simulink model "ACC"  (R2025b)
settings: Solver=VariableStepAuto  StartTime=0.0  StopTime=10.0  RelTol=1e-3
settings Model: DataDictionary=ACC.sldd  Creator=vmari  LastModifiedBy=spadhi

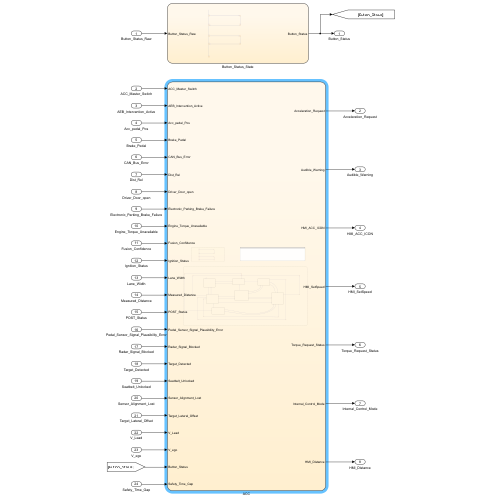
[thumbnail: Simulink's stored preview of the top-level diagram]
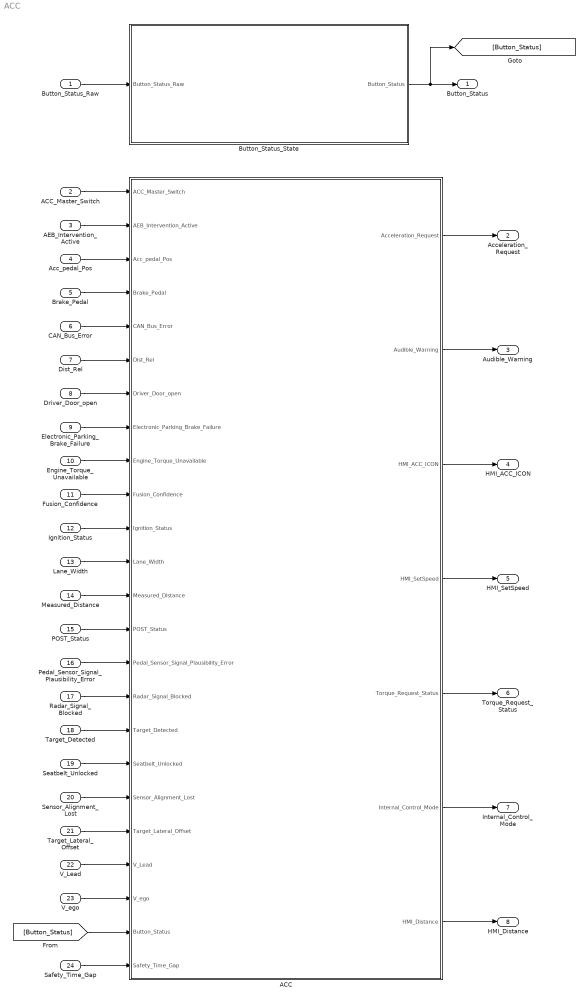
== system ACC ==
  Button_Status_Raw : Inport
  ACC_Master_Switch : Inport  Port=2
  AEB_Intervention_Active : Inport  Port=3
  Acc_pedal_Pos : Inport  Port=4
  Brake_Pedal : Inport  Port=5
  CAN_Bus_Error : Inport  Port=6
  Dist_Rel : Inport  Port=7
  Driver_Door_open : Inport  Port=8
  Electronic_Parking_Brake_Failure : Inport  Port=9
  Engine_Torque_Unavailable : Inport  Port=10
  Fusion_Confidence : Inport  Port=11
  Ignition_Status : Inport  Port=12
  Lane_Width : Inport  Port=13
  Measured_Distance : Inport  Port=14
  POST_Status : Inport  Port=15
  Pedal_Sensor_Signal_Plausibility_Error : Inport  Port=16
  Radar_Signal_Blocked : Inport  Port=17
  Target_Detected : Inport  Port=18
  Seatbelt_Unlocked : Inport  Port=19
  Sensor_Alignment_Lost : Inport  Port=20
  Target_Lateral_Offset : Inport  Port=21
  V_Lead : Inport  Port=22
  V_ego : Inport  Port=23
  Safety_Time_Gap : Inport  Port=24
  ACC : Stateflow chart  TreatAsAtomicUnit=on
  Button_Status_State : Stateflow chart  TreatAsAtomicUnit=on
  Button_Status : Outport
  Acceleration_Request : Outport  Port=2
  Audible_Warning : Outport  Port=3
  HMI_ACC_ICON : Outport  Port=4
  HMI_SetSpeed : Outport  Port=5
  Torque_Request_Status : Outport  Port=6
  Internal_Control_Mode : Outport  Port=7
  HMI_Distance : Outport  Port=8
  wires:
  Button_Status_Raw/1 -> Button_Status_State/1(Button_Status_Raw)
  Button_Status_State/1(Button_Status) -> [Button_Status], Button_Status/1
  [Button_Status] -> ACC/23(Button_Status)
  ACC_Master_Switch/1 -> ACC/1(ACC_Master_Switch)
  AEB_Intervention_Active/1 -> ACC/2(AEB_Intervention_Active)
  Acc_pedal_Pos/1 -> ACC/3(Acc_pedal_Pos)
  Brake_Pedal/1 -> ACC/4(Brake_Pedal)
  CAN_Bus_Error/1 -> ACC/5(CAN_Bus_Error)
  Driver_Door_open/1 -> ACC/7(Driver_Door_open)
  Electronic_Parking_Brake_Failure/1 -> ACC/8(Electronic_Parking_Brake_Failure)
  Engine_Torque_Unavailable/1 -> ACC/9(Engine_Torque_Unavailable)
  Fusion_Confidence/1 -> ACC/10(Fusion_Confidence)
  Ignition_Status/1 -> ACC/11(Ignition_Status)
  Dist_Rel/1 -> ACC/6(Dist_Rel)
  Lane_Width/1 -> ACC/12(Lane_Width)
  Measured_Distance/1 -> ACC/13(Measured_Distance)
  POST_Status/1 -> ACC/14(POST_Status)
  Pedal_Sensor_Signal_Plausibility_Error/1 -> ACC/15(Pedal_Sensor_Signal_Plausibility_Error)
  Radar_Signal_Blocked/1 -> ACC/16(Radar_Signal_Blocked)
  Target_Detected/1 -> ACC/17(Target_Detected)
  Seatbelt_Unlocked/1 -> ACC/18(Seatbelt_Unlocked)
  Sensor_Alignment_Lost/1 -> ACC/19(Sensor_Alignment_Lost)
  Target_Lateral_Offset/1 -> ACC/20(Target_Lateral_Offset)
  Safety_Time_Gap/1 -> ACC/24(Safety_Time_Gap)
  V_ego/1 -> ACC/22(V_ego)
  V_Lead/1 -> ACC/21(V_Lead)
  ACC/1(Acceleration_Request) -> Acceleration_Request/1
  ACC/2(Audible_Warning) -> Audible_Warning/1
  ACC/3(HMI_ACC_ICON) -> HMI_ACC_ICON/1
  ACC/4(HMI_SetSpeed) -> HMI_SetSpeed/1
  ACC/5(Torque_Request_Status) -> Torque_Request_Status/1
  ACC/6(Internal_Control_Mode) -> Internal_Control_Mode/1
  ACC/7(HMI_Distance) -> HMI_Distance/1

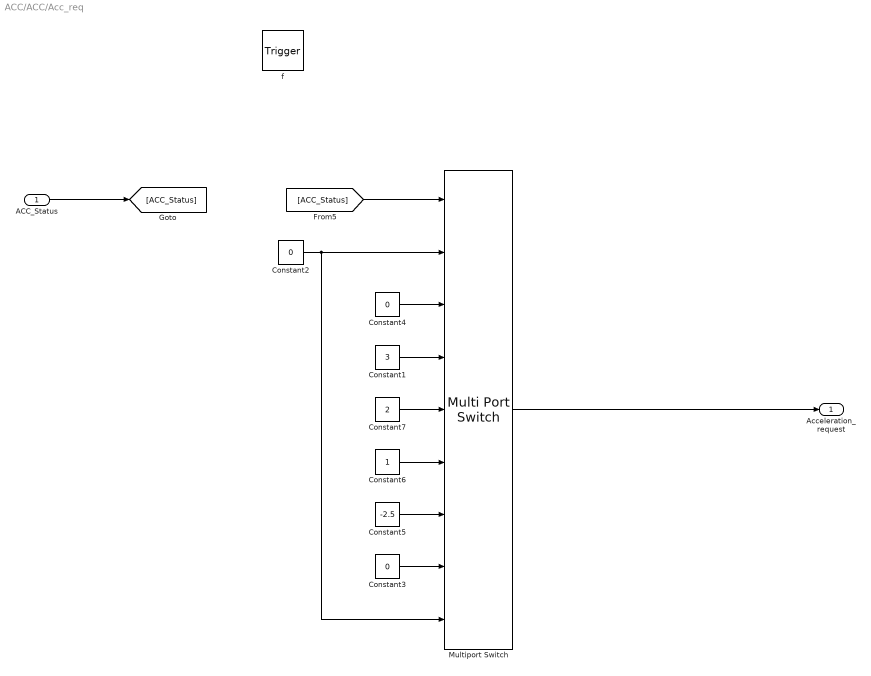
== system ACC/ACC/Acc_req ==
  ACC_Status : Inport  OutDataTypeStr=double  PortDimensions=1
  f : TriggerPort  TriggerType=function-call  VariantControl=(inherit)  SampleTime=0.01
      settings: CopyFcn=Stateflow.SLINSF.SimulinkMan.removeBlockPreDeleteFcn  PreDeleteFcn=Stateflow.SLINSF.SimulinkMan.unsafePredeleteFcn
  Constant1 : Constant  Value=3
  Constant2 : Constant  Value=0
  Constant3 : Constant  Value=0
  Constant4 : Constant  Value=0
  Constant5 : Constant  Value=-2.5
  Constant6 : Constant
  Constant7 : Constant  Value=2
  Multiport Switch : MultiPortSwitch  DataPortOrder=Zero-based contiguous  Inputs=7  DataPortForDefault=Additional data port  zeroidx=on  SaturateOnIntegerOverflow=off  InputSameDT=off
  Acceleration_request : Outport
  wires:
  ACC_Status/1 -> [ACC_Status]
  [ACC_Status] -> Multiport Switch/1
  Constant2/1 -> Multiport Switch/9, Multiport Switch/2
  Constant3/1 -> Multiport Switch/8
  Constant4/1 -> Multiport Switch/3
  Constant5/1 -> Multiport Switch/7
  Multiport Switch/1 -> Acceleration_request/1
  Constant1/1 -> Multiport Switch/4
  Constant7/1 -> Multiport Switch/5
  Constant6/1 -> Multiport Switch/6

== stateflow chart ACC/Button_Status_State ==
  (default) -> (junction 29)
  (junction 29) -> (junction 4) [order 1] : [Button_Status_Raw == 1]
  (junction 29) -> (junction 8) [order 2]
  (junction 4) -> (junction 6) : {Button_Status = Dt_Enum_Button_Status_E.SET}
  (junction 6) -> (junction 8)
  (junction 8) -> (junction 11)
  (junction 11) -> (junction 13) [order 1] : [Button_Status_Raw == 2]
  (junction 11) -> (junction 17) [order 2]
  (junction 13) -> (junction 15) : {Button_Status = Dt_Enum_Button_Status_E.CANCEL}
  (junction 15) -> (junction 17)
  (junction 17) -> (junction 20) : {Button_Status = Dt_Enum_Button_Status_E.NONE}
  data: Button_Status_Raw input; Button_Status output Enum: Dt_Enum_Button_Status_E

== stateflow chart ACC/ACC ==
  state Set_Speed_Controller [parallel]
    settings: executionOrder=2
    (default) -> (junction 162)
    (junction 162) -> (junction 165) [order 1] : [Target_Detected == true]
    (junction 162) -> (junction 164) [order 2]
    (junction 165) -> (junction 168) : {V_set = V_Lead}
    (junction 168) -> (junction 164)
    (junction 164) -> (junction 171)
    (junction 171) -> (junction 173) [order 1] : [Target_Detected == false && Button_Status ==Dt_Enum_Button_Status_E.SET ]
    (junction 171) -> (junction 176) [order 2]
    (junction 173) -> (junction 175) : {V_set = V_ego}
    (junction 175) -> (junction 176)
  state Acceleration_request = Acc_req(ACC_Status) [function]
  state ACC_States [parallel]
    settings: executionOrder=1
    state ACC_Off
      en:
      ACC_Status = 0;
      du:
      Acceleration_Request = Acc_req(ACC_Status);
      Torque_Request_Status = Disabled;
      HMI_ACC_ICON = Off;
      HMI_SetSpeed = V_set;
      Audible_Warning = None;
      Internal_Control_Mode = Standstill;
    state ACC_Fault
      ACC_Status = 2;
      Acceleration_Request = Acc_req(ACC_Status);
      %Rampto0
      Torque_Request_Status = Fault;
      HMI_ACC_ICON = Red;
      Audible_Warning = Loud_Chime;
      Internal_Control_Mode = Error;
    state ACC_Override
      en:
      ACC_Status = 6;
      du:
      Acceleration_Request = Acc_req(ACC_Status);
      Torque_Request_Status = Override;
      HMI_ACC_ICON = Blink_Green;
      Audible_Warning = Chime;%V>Vset for x
      Internal_Control_Mode = Passive;
    state ACC_Active
      ACC_Status = 3;
      Acceleration_Request = Acc_req(ACC_Status);
      %Vset-Vego
      Torque_Request_Status = Longi;
      HMI_ACC_ICON = Green;
      HMI_SetSpeed = 0;%Current_SetSpeed
      Audible_Warning = Single_Beep;
      Internal_Control_Mode = Speedctrl;
    state ACC_Active_Follow
      ACC_Status = 4;
      Acceleration_Request = Acc_req(ACC_Status);
      %Drel Cal
      Torque_Request_Status = Dis_active;
      HMI_ACC_ICON = Green;
      HMI_Distance = 1;%1-5 Bars
      Audible_Warning = None;
      Internal_Control_Mode = Distctrl;
    state ACC_Stanby
      en:
      ACC_Status = 1;
      du:
      Acceleration_Request = Acc_req(ACC_Status);
      Torque_Request_Status = Standby;
      HMI_ACC_ICON = White;
      HMI_SetSpeed = 0;%Prev Speed
      Audible_Warning = None;
      Internal_Control_Mode = Monitoring;
    state ACC_Stop_Hold
      en:
      ACC_Status = 5;
      du:
      Acceleration_Request = Acc_req(ACC_Status);
      Torque_Request_Status = Hold_Req;
      HMI_ACC_ICON = Green;
      Audible_Warning = None;
      Internal_Control_Mode = Standstill;
    (junction 371) -> (junction 378)
    (junction 384) -> (junction 371)
    (junction 378) -> (junction 373)
    (junction 383) -> (junction 373)
    (junction 374) -> (junction 373)
    (junction 373) -> ACC_Fault
    (junction 380) -> (junction 374)
    (junction 386) -> (junction 383) : [CAN_Bus_Error == true ||...
        | Sensor_Alignment_Lost == true]
    (default) -> ACC_Off
    ACC_Override -> (junction 375) [order 3] : [Brake_Pedal == Dt_Enum_Pedal_E.PRESSED || ...
        | Button_Status == Dt_Enum_Button_Status_E.CANCEL]
    (junction 375) -> (junction 425) : [Brake_Pedal == Dt_Enum_Pedal_E.PRESSED ||Button_Status == Dt_Enum_Button_Status_E.CANCEL]
    ACC_Override -> ACC_Fault [order 4] : [Pedal_Sensor_Signal_Plausibility_Error == true  ]
    ACC_Off -> ACC_Fault [order 2] : [Ignition_Status == Dt_Enum_Ignition_Status_E.RUN &&...
        | ACC_Master_Switch == Dt_Enum_ACC_Master_Switch_E.ON &&...
        | POST_Status == Dt_Enum_POST_Status_E.FAILED]
    ACC_Override -> ACC_Active_Follow [order 1] : [Acc_pedal_Pos < 5 && Target_Detected == true]
    ACC_Fault -> ACC_Off : [Ignition_Status == Dt_Enum_Ignition_Status_E.OFF ||...
        | ACC_Master_Switch == Dt_Enum_ACC_Master_Switch_E.OFF]
    ACC_Active -> ACC_Fault [order 4] : [Radar_Signal_Blocked == true || ...
        | Engine_Torque_Unavailable == true]
    ACC_Active_Follow -> ACC_Override [order 3] : [Acc_pedal_Pos > 15]
    ACC_Override -> ACC_Active [order 2] : [Acc_pedal_Pos < 5 && Target_Detected == false]
    ACC_Active -> ACC_Override [order 1] : [Acc_pedal_Pos > 15]
    ACC_Off -> ACC_Stanby [order 1] : [Ignition_Status == Dt_Enum_Ignition_Status_E.RUN &&...
        | ACC_Master_Switch == Dt_Enum_ACC_Master_Switch_E.ON &&...
        | POST_Status == Dt_Enum_POST_Status_E.SUCCESS]
    ACC_Stanby -> ACC_Off [order 3] : [Ignition_Status == Dt_Enum_Ignition_Status_E.OFF ||...
        | ACC_Master_Switch == Dt_Enum_ACC_Master_Switch_E.OFF]
    ACC_Active_Follow -> (junction 380) [order 5] : [Fusion_Confidence < 40 || AEB_Intervention_Active == true]
    ACC_Stanby -> (junction 386) [order 4]
    ACC_Active -> ACC_Stanby [order 3] : [Button_Status == Dt_Enum_Button_Status_E.CANCEL]
    (junction 381) -> ACC_Stanby
    ACC_Active -> ACC_Active_Follow [order 2] : [Target_Detected == true &&...
        |  Measured_Distance < Safety_Time_Gap]
    (junction 408) -> (junction 381)
    ACC_Stanby -> ACC_Active [order 2] : [Button_Status == Dt_Enum_Button_Status_E.SET&& ...
        | V_ego >= 30 && ...
        | Brake_Pedal == Dt_Enum_Pedal_E.RELEASED && ...
        | Target_Detected == false]
    ACC_Active_Follow -> ACC_Active [order 1] : [Target_Detected == true ||...
        | Target_Lateral_Offset > Lane_Width]
    (junction 382) -> ACC_Stanby
    (junction 421) -> (junction 382)
    ACC_Stanby -> ACC_Active_Follow [order 1] : [Button_Status == Dt_Enum_Button_Status_E.SET && ...
        | V_ego >= 30 && ...
        | Brake_Pedal == Dt_Enum_Pedal_E.RELEASED && ...
        | Target_Detected == true]
    ACC_Stop_Hold -> ACC_Stanby [order 2] : [Driver_Door_open == true || ...
        | Seatbelt_Unlocked == true || ...
        | Brake_Pedal == Dt_Enum_Pedal_E.PRESSED]
    ACC_Active_Follow -> ACC_Stop_Hold [order 2] : [V_ego < 1 && V_Lead == 0 && Dist_Rel < 3.5]
    ACC_Stop_Hold -> ACC_Active_Follow [order 1] : [V_ego < 1 && V_Lead == 0 && Dist_Rel < 3.5]
    ACC_Active_Follow -> (junction 397) [order 4] : [Brake_Pedal == Dt_Enum_Pedal_E.PRESSED || Button_Status == Dt_Enum_Button_Status_E.CANCEL]
    ACC_Stop_Hold -> (junction 384) [order 3] : [Electronic_Parking_Brake_Failure == true]
    (junction 397) -> (junction 421)
    (junction 425) -> (junction 408)
  data: ACC_Status function_input double size=1; Acceleration_request function_output; ACC_Master_Switch input; AEB_Intervention_Active input; Acc_pedal_Pos input; Brake_Pedal input; CAN_Bus_Error input; Dist_Rel input; Driver_Door_open input; Electronic_Parking_Brake_Failure input; Engine_Torque_Unavailable input; Fusion_Confidence input; Ignition_Status input; Lane_Width input; Measured_Distance input; POST_Status input; Pedal_Sensor_Signal_Plausibility_Error input; Radar_Signal_Blocked input; Target_Detected input; Seatbelt_Unlocked input; Sensor_Alignment_Lost input; Target_Lateral_Offset input; V_Lead input; V_ego input; Button_Status input; Safety_Time_Gap input double; Acceleration_Request output; Audible_Warning output Enum: Dt_Enum_Audible_Warning_E; HMI_ACC_ICON output Enum: Dt_Enum_HMI_ACC_ICON_E; HMI_SetSpeed output; Torque_Request_Status output Enum: Dt_Enum_Torque_Request_Status_E; Internal_Control_Mode output Enum: Dt_Enum_Internal_Control_Mode_E; HMI_Distance output; ACC_Status local; V_set local
